simulink model "BenchmarkTestHarness"  (R2019b)
settings: Solver=FixedStepAuto  StartTime=0.0  StopTime=1000  FixedStep=0.01  RelTol=1e-3
values from neighbouring files (symbols this model uses):
  dtSim = 0.01    [RunBenchmarkTests.m]
undefined symbols (not defined in the file or in its folder): OP
settings Model: PauseTimes=1  Creator=tarek  LastModifiedBy=tarek
settings DebuggingCC: UnconnectedInputMsg=none  UnconnectedOutputMsg=none  UnconnectedLineMsg=none
settings ModelReferenceCC: EnableRefExpFcnMdlSchedulingChecks=off
settings RTWCC: Description=Generic Real-Time Target

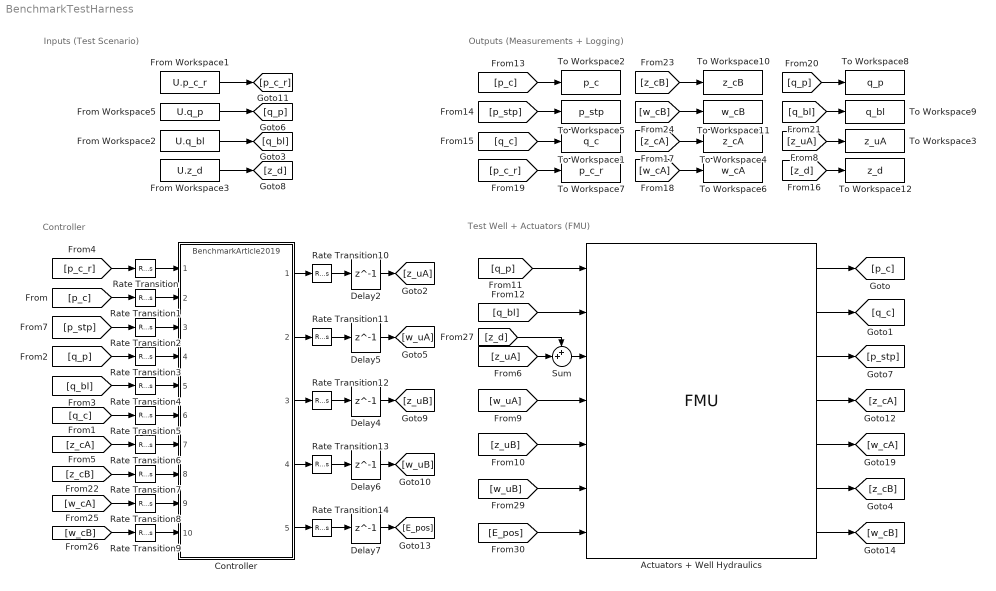
== system BenchmarkTestHarness ==
  note: Inputs (Test Scenario)
  note: Test Well + Actuators (FMU)
  note: Controller
  note: Outputs (Measurements + Logging)
  Actuators + Well Hydraulics : FMU  FMUName=SelectedFMU.fmu  FMUMode=CoSimulation
      mask Type: ActuatorAndWellHydraulics_TestHarness [Co-Simulation, v2.0]
      mask Display:
      | disp('ActuatorAndWellHydraulics_TestHarness');
      | port_label('output',1,'p_c');
      | port_label('output',2,'q_c');
      | port_label('output',3,'p_stp');
      | port_label('output',4,'z_cA');
      | port_label('output',5,'w_cA');
      | port_label('output',6,'z_cB');
      | port_label('output',7,'w_cB');
      | port_label('input',1,'q_p');
      | port_label('input',2,'q_bl');
      | port_label('input',3,'z_uA');
      | port_label('input',4,'w_uA');
      | port_label('input',5,'z_uB');
      | port_label('input',6,'w_uB');
      | port_label('input',7,'E_ctrl_pos');
  Controller : ModelReference  ModelNameDialog=BenchmarkArticle2019  SimulationMode=Normal  ModelReferenceVersion=1.1
  Delay2 : Delay  DelayLength=1  InitialCondition=OP.z_c0(1)
  Delay4 : Delay  DelayLength=1  InitialCondition=OP.z_c0(2)
  Delay5 : Delay  DelayLength=1  InitialCondition=0
  Delay6 : Delay  DelayLength=1  InitialCondition=0
  Delay7 : Delay  DelayLength=1  InitialCondition=0
  From Workspace1 : FromWorkspace  VariableName=U.p_c_r  SampleTime=dtSim  OutputAfterFinalValue=Holding final value
  From Workspace2 : FromWorkspace  VariableName=U.q_bl  SampleTime=dtSim  OutputAfterFinalValue=Holding final value
  From Workspace3 : FromWorkspace  VariableName=U.z_d  SampleTime=dtSim  OutputAfterFinalValue=Holding final value
  From Workspace5 : FromWorkspace  VariableName=U.q_p  SampleTime=dtSim  OutputAfterFinalValue=Holding final value
  Rate Transition{,1..14} (15 alike) : RateTransition
  Sum : Sum  Inputs=++|
  To Workspace1 : ToWorkspace  VariableName=q_c  SaveFormat=Timeseries  SampleTime=-1
  To Workspace10 : ToWorkspace  VariableName=z_cB  SaveFormat=Timeseries  SampleTime=-1
  To Workspace11 : ToWorkspace  VariableName=w_cB  SaveFormat=Timeseries  SampleTime=-1
  To Workspace12 : ToWorkspace  VariableName=z_d  SaveFormat=Timeseries  SampleTime=-1
  To Workspace2 : ToWorkspace  VariableName=p_c  SaveFormat=Timeseries  SampleTime=-1
  To Workspace3 : ToWorkspace  VariableName=z_uA  SaveFormat=Timeseries  SampleTime=-1
  To Workspace4 : ToWorkspace  VariableName=z_cA  SaveFormat=Timeseries  SampleTime=-1
  To Workspace5 : ToWorkspace  VariableName=p_stp  SaveFormat=Timeseries  SampleTime=-1
  To Workspace6 : ToWorkspace  VariableName=w_cA  SaveFormat=Timeseries  SampleTime=-1
  To Workspace7 : ToWorkspace  VariableName=p_c_r  SaveFormat=Timeseries  SampleTime=-1
  To Workspace8 : ToWorkspace  VariableName=q_p  SaveFormat=Timeseries  SampleTime=-1
  To Workspace9 : ToWorkspace  VariableName=q_bl  SaveFormat=Timeseries  SampleTime=-1
  wires:
  [q_p] -> Actuators + Well Hydraulics/1
  [q_bl] -> Actuators + Well Hydraulics/2
  Actuators + Well Hydraulics/1 -> [p_c]
  Actuators + Well Hydraulics/2 -> [q_c]
  [z_uA] -> Sum/2
  Actuators + Well Hydraulics/3 -> [p_stp]
  Actuators + Well Hydraulics/4 -> [z_cA]
  From Workspace2/1 -> [q_bl]
  From Workspace5/1 -> [q_p]
  From Workspace1/1 -> [p_c_r]
  [p_c] -> To Workspace2/1
  [p_stp] -> To Workspace5/1
  [q_c] -> To Workspace1/1
  [z_cA] -> To Workspace4/1
  [w_cA] -> To Workspace6/1
  [p_c_r] -> To Workspace7/1
  [q_p] -> To Workspace8/1
  [q_bl] -> To Workspace9/1
  Controller/1 -> Rate Transition10/1
  Controller/3 -> Rate Transition12/1
  Controller/4 -> Rate Transition13/1
  Actuators + Well Hydraulics/5 -> [w_cA]
  Actuators + Well Hydraulics/6 -> [z_cB]
  [w_uA] -> Actuators + Well Hydraulics/4
  [z_uB] -> Actuators + Well Hydraulics/5
  [w_uB] -> Actuators + Well Hydraulics/6
  [E_pos] -> Actuators + Well Hydraulics/7
  Delay2/1 -> [z_uA]
  Delay4/1 -> [z_uB]
  Delay5/1 -> [w_uA]
  Delay6/1 -> [w_uB]
  Delay7/1 -> [E_pos]
  Actuators + Well Hydraulics/7 -> [w_cB]
  [z_cB] -> To Workspace10/1
  [w_cB] -> To Workspace11/1
  Controller/5 -> Rate Transition14/1
  Controller/2 -> Rate Transition11/1
  [p_c] -> Rate Transition1/1
  [p_c_r] -> Rate Transition/1
  [p_stp] -> Rate Transition2/1
  [q_p] -> Rate Transition3/1
  [q_bl] -> Rate Transition4/1
  [q_c] -> Rate Transition5/1
  [z_cA] -> Rate Transition6/1
  [z_cB] -> Rate Transition7/1
  [w_cA] -> Rate Transition8/1
  [w_cB] -> Rate Transition9/1
  Rate Transition/1 -> Controller/1
  Rate Transition1/1 -> Controller/2
  Rate Transition2/1 -> Controller/3
  Rate Transition3/1 -> Controller/4
  Rate Transition4/1 -> Controller/5
  Rate Transition5/1 -> Controller/6
  Rate Transition6/1 -> Controller/7
  Rate Transition7/1 -> Controller/8
  Rate Transition8/1 -> Controller/9
  Rate Transition9/1 -> Controller/10
  Rate Transition10/1 -> Delay2/1
  Rate Transition11/1 -> Delay5/1
  Rate Transition12/1 -> Delay4/1
  Rate Transition13/1 -> Delay6/1
  Rate Transition14/1 -> Delay7/1
  From Workspace3/1 -> [z_d]
  [z_uA] -> To Workspace3/1
  [z_d] -> To Workspace12/1
  Sum/1 -> Actuators + Well Hydraulics/3
  [z_d] -> Sum/1
